simulink model "fir_filter_example_org"  (Simulink 10.0)
settings: Solver=FixedStepDiscrete  StartTime=0.0  StopTime=300  RelTol=1e-3
PostLoadFcn:
  | Fpass = 0.45;  % Passband Frequency
  | Fstop = 0.55;  % Stopband Frequency
  | Apass = 1;     % Passband Ripple (dB)
  | Astop = 60;    % Stopband Attenuation (dB)
  | 
  | h = fdesign.lowpass('fp,fst,ap,ast', Fpass, Fstop, Apass, Astop);
  | 
  | Hd = design(h, 'equiripple', ...
  |     'FilterStructure', 'dfsymfir', ...
  |     'MinOrder', 'any', ...
  |     'StopbandShape', 'flat');
  | 
  | T = 300;
undefined symbols (not defined in the file): chirp
libraries: hdlsllib x2, dspsrcs4 x1, simulink x1, simulink_need_slupdate x1
settings Model: DataTypeOverride=Off  Creator=cchung  LastModifiedBy=bhisma
settings DataIOCC: LimitDataPoints=on  SaveOutput=off  SaveTime=off
settings OptimizationCC: BlockReduction=off  ConditionallyExecuteInputs=off  DefaultParameterBehavior=Inlined
settings DebuggingCC: AlgebraicLoopMsg=error  UnderspecifiedInitializationDetection=Simplified  MergeDetectMultiDrivingBlocksExec=error  SolverPrmCheckMsg=warning  SingleTaskRateTransMsg=error
settings HardwareCC: ProdHWDeviceType=ASIC/FPGA->ASIC/FPGA  ProdEqTarget=off
settings GRTTargetCC: GeneratePreprocessorConditionals=Disable all  CombineOutputUpdateFcns=on  GRTInterface=off
settings ConfigComp: CovExternalEMLEnable=off  CovSFcnEnable=off

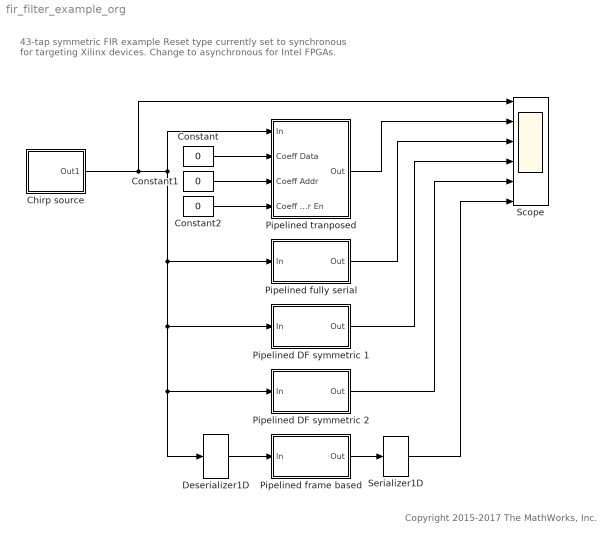
== system fir_filter_example_org ==
  note: Copyright 2015-2017 The MathWorks, Inc.
  note: 43-tap symmetric FIR example
      |
      | Reset type currently set to synchronous for targeting Xilinx devices.
      | Change to asynchronous for Intel FPGAs.
  Chirp source : Subsystem
  Constant : Constant  Value=0  OutDataTypeStr=fixdt(1,16,15)  SampleTime=-1
  Constant1 : Constant  Value=0  OutDataTypeStr=fixdt(0,8,0)  SampleTime=-1
  Constant2 : Constant  Value=0  OutDataTypeStr=boolean  SampleTime=-1
  Deserializer1D : hdlsllib/HDL Operations/Deserializer1D  Ratio=2  IdleCycles=0  InitialCondition=0  startIn=off  validIn=off  validOut=off  inputDataDimensions=-1  inputSampleTime=-1  inputSignalType=auto
      settings: SourceProductName=Simulink  SourceProductBaseCode=SL
  Pipelined DF symmetric 1 : Subsystem  Tag=BlockMethodSubSystem
  Pipelined DF symmetric 2 : Subsystem  Tag=BlockMethodSubSystem
  Pipelined frame based : Subsystem  Tag=BlockMethodSubSystem
  Pipelined fully serial : Subsystem  Tag=BlockMethodSubSystem
  Pipelined tranposed : Subsystem  Tag=BlockMethodSubSystem
  Scope : Scope  NumInputPorts=6
  Serializer1D : hdlsllib/HDL Operations/Serializer1D  Ratio=2  IdleCycles=0  validIn=off  startOut=off  validOut=off  inputDataDimensions=-1  inputSampleTime=-1  inputSignalType=auto
      settings: SourceProductName=Simulink  SourceProductBaseCode=SL
  wires:
  Pipelined tranposed/1(Out) -> Scope/2
  Chirp source/1(Out1) -> Scope/1, Pipelined tranposed/1(In), Deserializer1D/1, Pipelined DF symmetric 2/1(In), Pipelined DF symmetric 1/1(In), Pipelined fully serial/1(In)
  Pipelined fully serial/1(Out) -> Scope/3
  Pipelined DF symmetric 1/1(Out) -> Scope/4
  Pipelined DF symmetric 2/1(Out) -> Scope/5
  Constant/1 -> Pipelined tranposed/2(Coeff Data)
  Constant1/1 -> Pipelined tranposed/3(Coeff Addr)
  Constant2/1 -> Pipelined tranposed/4(Coeff Wr En)
  Serializer1D/1 -> Scope/6
  Deserializer1D/1 -> Pipelined frame based/1(In)
  Pipelined frame based/1(Out) -> Serializer1D/1

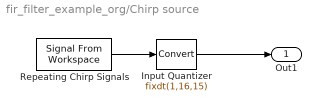
== system fir_filter_example_org/Chirp source ==
  Input Quantizer : DataTypeConversion  OutDataTypeStr=fixdt(1,16,15)  RndMeth=Round  SaturateOnIntegerOverflow=on
  Repeating Chirp Signals : dspsrcs4/Signal From Workspace  X=[chirp(0:T-1,0,T-1,0.4),chirp(0:T-1,0,T-1,0.4)]  Ts=1  nsamps=1  OutputAfterFinalValue=Setting to zero  ignoreOrWarnInputAndFrameLengths=off  OutputFrames=on
  Out1 : Outport
  wires:
  Input Quantizer/1 -> Out1/1
  Repeating Chirp Signals/1 -> Input Quantizer/1

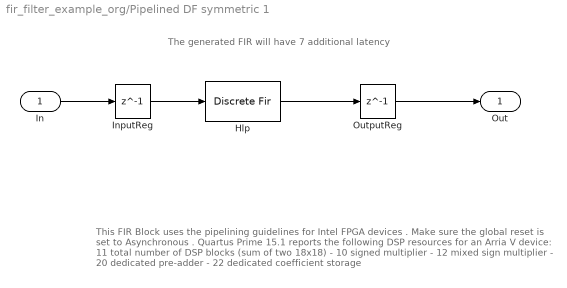
== system fir_filter_example_org/Pipelined DF symmetric 1 ==
  note: This FIR Block uses the pipelining guidelines for Intel FPGA devices .
      | Make sure the global reset is set to Asynchronous .
      |
      | Quartus Prime 15.1 reports the following DSP resources for an Arria V device:
      |
      | 11 total number of DSP blocks (sum of two 18x18)
      | - 10 signed multiplier
      | - 12 mixed sign multiplier
      | - 20 dedicated pre-adder
      | - 22 dedicated coefficient storage
  note: The generated FIR will have 7 additional latency
  In : Inport
  Hlp : DiscreteFir  Tag=BlockMethodSubSystem  FilterStructure=Direct form symmetric  Coefficients=Hd.Numerator
      settings: AttributesFormatString=|
      | AddPipelineRegisters : on
      | InputPipeline : 1
      | MultiplierOutputPipeline : 1
  InputReg : Delay  DelayLength=1  InitialCondition=0
  OutputReg : Delay  DelayLength=1  InitialCondition=0
  Out : Outport
  wires:
  InputReg/1 -> Hlp/1
  In/1 -> InputReg/1
  OutputReg/1 -> Out/1
  Hlp/1 -> OutputReg/1

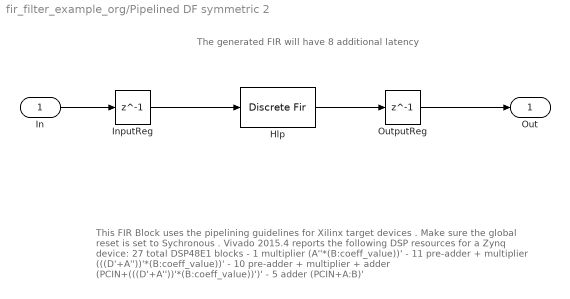
== system fir_filter_example_org/Pipelined DF symmetric 2 ==
  note: The generated FIR will have 8 additional latency
  note: This FIR Block uses the pipelining guidelines for Xilinx target devices .
      | Make sure the global reset is set to Sychronous .
      |
      | Vivado 2015.4 reports the following DSP resources for a Zynq device:
      |
      | 27 total DSP48E1 blocks
      | - 1 multiplier (A''*(B:coeff_value))'
      | - 11 pre-adder + multiplier (((D'+A''))'*(B:coeff_value))'
      | - 10 pre-adder + multiplier + adder (PCIN+(((D'+A''))'*(B:coeff_value))')'
      | - 5 adder (PCIN+A:B)'
  In : Inport
  Hlp : DiscreteFir  Tag=BlockMethodSubSystem  FilterStructure=Direct form symmetric  Coefficients=Hd.Numerator
      settings: AttributesFormatString=|
      | AddPipelineRegisters : on
      | InputPipeline : 1
      | MultiplierInputPipeline : 1
      | MultiplierOutputPipeline : 1
  InputReg : Delay  DelayLength=1  InitialCondition=0
  OutputReg : Delay  DelayLength=1  InitialCondition=0
  Out : Outport
  wires:
  Hlp/1 -> OutputReg/1
  OutputReg/1 -> Out/1
  In/1 -> InputReg/1
  InputReg/1 -> Hlp/1

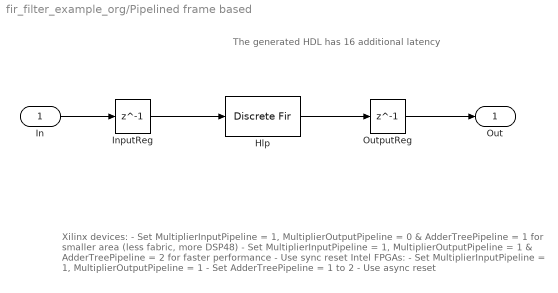
== system fir_filter_example_org/Pipelined frame based ==
  note: The generated HDL has 16 additional latency
  note: Xilinx devices:
      | - Set MultiplierInputPipeline = 1, MultiplierOutputPipeline = 0 & AdderTreePipeline = 1
      | for smaller area (less fabric, more DSP48)
      | - Set MultiplierInputPipeline = 1, MultiplierOutputPipeline = 1 & AdderTreePipeline = 2
      | for faster performance
      | - Use sync reset
      |
      | Intel FPGAs:
      | - Set MultiplierInputPipeline = 1, MultiplierOutputPipeline = 1
      | - Set AdderTreePipeline = 1 to 2
      | - Use async reset
  In : Inport
  Hlp : DiscreteFir  Tag=BlockMethodSubSystem  Coefficients=Hd.Numerator  InputProcessing=Columns as channels (frame based)
      settings: AttributesFormatString=|
      | Architecture : Frame Based
      | AdderTreePipeline : 2
      | MultiplierInputPipeline : 1
      | MultiplierOutputPipeline : 1
  InputReg : Delay  DelayLength=1  InitialCondition=0
  OutputReg : Delay  DelayLength=1  InitialCondition=0
  Out : Outport
  wires:
  InputReg/1 -> Hlp/1
  In/1 -> InputReg/1
  OutputReg/1 -> Out/1
  Hlp/1 -> OutputReg/1

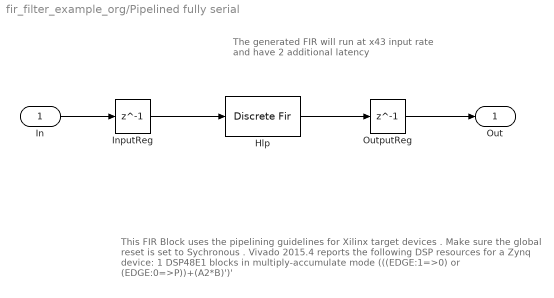
== system fir_filter_example_org/Pipelined fully serial ==
  note: The generated FIR will run at x43 input rate
      | and have 2 additional latency
  note: This FIR Block uses the pipelining guidelines for Xilinx target devices .
      | Make sure the global reset is set to Sychronous .
      |
      | Vivado 2015.4 reports the following DSP resources for a Zynq device:
      |
      | 1 DSP48E1 blocks in multiply-accumulate mode
      | (((EDGE:1=>0) or (EDGE:0=>P))+(A2*B)')'
  In : Inport
  Hlp : DiscreteFir  Tag=BlockMethodSubSystem  Coefficients=Hd.Numerator
      settings: AttributesFormatString=|
      | Architecture : Fully Serial
      | MultiplierInputPipeline : 1
      | MultiplierOutputPipeline : 1
  InputReg : Delay  DelayLength=1  InitialCondition=0
  OutputReg : Delay  DelayLength=1  InitialCondition=0
  Out : Outport
  wires:
  InputReg/1 -> Hlp/1
  In/1 -> InputReg/1
  OutputReg/1 -> Out/1
  Hlp/1 -> OutputReg/1

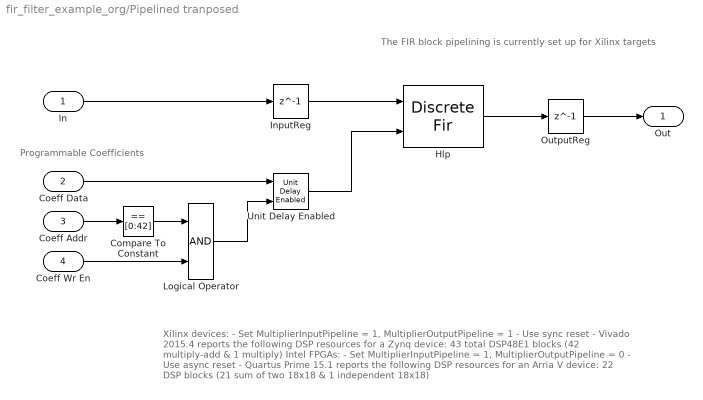
== system fir_filter_example_org/Pipelined tranposed ==
  note: Programmable Coefficients
  note: Xilinx devices:
      | - Set MultiplierInputPipeline = 1, MultiplierOutputPipeline = 1
      | - Use sync reset
      |
      | - Vivado 2015.4 reports the following DSP resources for a Zynq device:
      | 43 total DSP48E1 blocks (42 multiply-add & 1 multiply)
      |
      | Intel FPGAs:
      | - Set MultiplierInputPipeline = 1, MultiplierOutputPipeline = 0
      | - Use async reset
      |
      | - Quartus Prime 15.1 reports the following DSP resources for an Arria V device:
      | 22 DSP blocks (21 sum of two 18x18 & 1 independent 18x18)
  note: The FIR block pipelining is currently set up for Xilinx targets
  In : Inport
  Coeff Data : Inport  Port=2
  Coeff Addr : Inport  Port=3
  Coeff Wr En : Inport  Port=4
  Compare To Constant : simulink/Logic and Bit Operations/Compare To Constant  relop===  const=[0:42]  OutDataTypeStr=boolean
  Hlp : DiscreteFir  Tag=BlockMethodSubSystem  CoefSource=Input port  FilterStructure=Direct form transposed  Coefficients=Hd.Numerator
      settings: InputPortMap=u0,u1
      settings: AttributesFormatString=|
      | Architecture : Fully Parallel
      | MultiplierInputPipeline : 1
      | MultiplierOutputPipeline : 1
  InputReg : Delay  DelayLength=1  InitialCondition=0
  Logical Operator : Logic  AllPortsSameDT=off  OutDataTypeStr=boolean
  OutputReg : Delay  DelayLength=1  InitialCondition=0
  Unit Delay Enabled : simulink_need_slupdate/Unit Delay Enabled  vinit=Hd.Numerator  tsamp=-1
      settings: SourceProductName=Simulink  SourceProductBaseCode=SL
  Out : Outport
  wires:
  Hlp/1 -> OutputReg/1
  OutputReg/1 -> Out/1
  In/1 -> InputReg/1
  InputReg/1 -> Hlp/1
  Unit Delay Enabled/1 -> Hlp/2
  Coeff Data/1 -> Unit Delay Enabled/1
  Coeff Addr/1 -> Compare To Constant/1
  Compare To Constant/1 -> Logical Operator/1
  Coeff Wr En/1 -> Logical Operator/2
  Logical Operator/1 -> Unit Delay Enabled/2
